simulink model "Symulacja_URA_na_podstawie_aktualnego_TP"  (R2022b)
settings: Solver=VariableStepAuto  StartTime=0.0  StopTime=100  RelTol=1e-3
values from neighbouring files (symbols this model uses):
  TPP = 0.5    [TPP_change.m]
  Ts = TS    [PID_init.m]    (also in Plik_inicjalizujacy_symulacje_predyktora_Smitha.m = 0.01)
undefined symbols (not defined in the file or in its folder): DiscIntNeverNeededParam
settings Model: Creator=hpiet  LastModifiedBy=hpiet
settings DebuggingCC: UnderSpecifiedDimensionMsg=warning

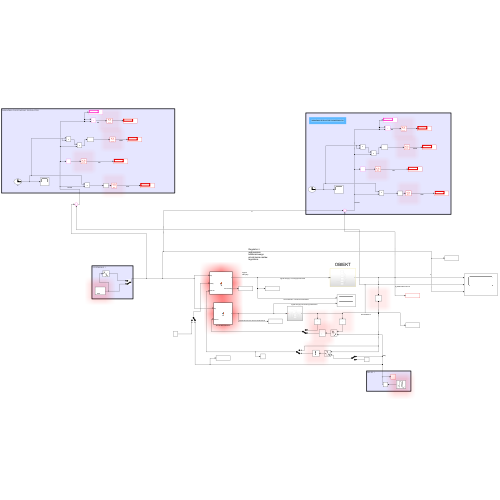
[thumbnail: Simulink's stored preview of the top-level diagram]
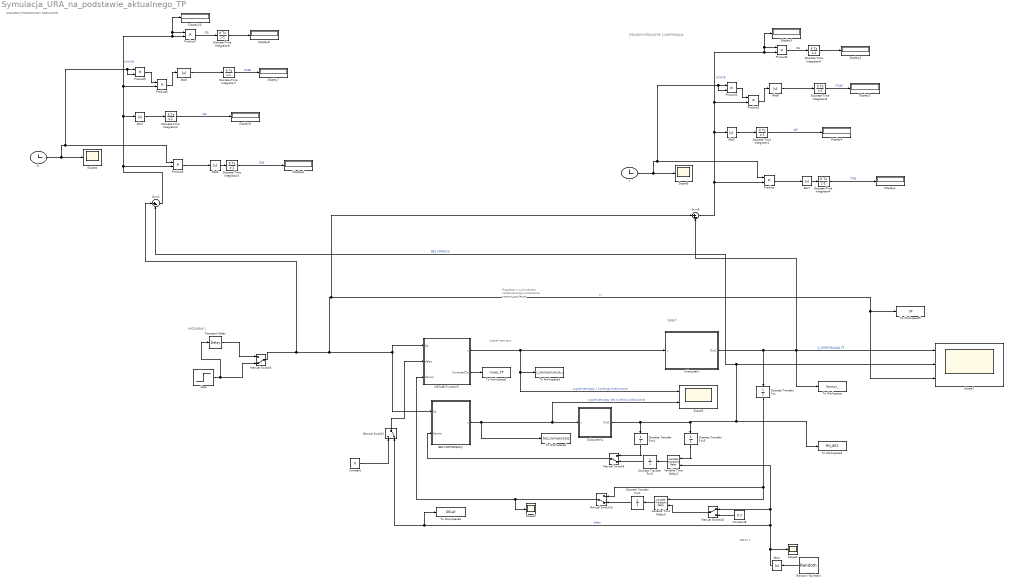
== system Symulacja_URA_na_podstawie_aktualnego_TP ==
  note: WSKAZNIKI REGULATOR Z KOMPENSACJA
  note: WSKAŹNIKI PODSTAWOWY REGULATOR
  note: OBIEKT
  note: DELAY 1
  note: sygnał sterujacy
  note: Regulator z wykonaniem każdorazowego przeliczenia nastaw regulatora
  note: OPÓŹNIENIE 1
  Abs{1..5,7..8} (7 alike) : Abs  SaturateOnIntegerOverflow=off
  BEZ KOMPENSACJI : MATLAB Function  TreatAsAtomicUnit=on  SystemSampleTime=TPP
  Constant : Constant  Value=0
  Constant8 : Constant  Value=0.3
  Discrete Transfer Fcn{,1..4} (5 alike) : DiscreteTransferFcn  Denominator=[1]  SampleTime=TPP
  Discrete-Time Integrator{1..8} (8 alike) : DiscreteIntegrator  SampleTime=Ts  ICPrevOutput=DiscIntNeverNeededParam  ICPrevScaledInput=DiscIntNeverNeededParam
  Display{1..10} (10 alike) : Display
  MATLAB Function3 : MATLAB Function  TreatAsAtomicUnit=on  SystemSampleTime=TPP
  Manual Switch{1,5..6,13} (4 alike) : ManualSwitch  CurrentSetting=0
  Manual Switch16 : ManualSwitch
  Product{,1..7} (8 alike) : Product
  Random Number1 : RandomNumber  Mean=1  Variance=0.0001  SampleTime=TPP
  Scope{1..2,4..5} (4 alike) : Scope
  Scope3 : Scope  NumInputPorts=2
  Scope7 : Scope  NumInputPorts=3
  Step : Step  Time=0  After=25  SampleTime=TPP
  Subsystem : Subsystem
  Subsystem1 : Subsystem
  Sum1 : Sum  Inputs=|+-
  Sum9 : Sum  Inputs=|+-
  To Workspace : ToWorkspace  VariableName=Sensor_  SaveFormat=Timeseries  SampleTime=-1
  To Workspace1 : ToWorkspace  VariableName=nowe_TP  SaveFormat=Timeseries  SampleTime=-1
  To Workspace2 : ToWorkspace  VariableName=PID_BEZ  SaveFormat=Timeseries  SampleTime=-1
  To Workspace3 : ToWorkspace  VariableName=z_kompensacja_u  SaveFormat=Timeseries  SampleTime=-1
  To Workspace4 : ToWorkspace  VariableName=bez_kompensacji  SaveFormat=Timeseries  SampleTime=-1
  To Workspace5 : ToWorkspace  VariableName=SP  SaveFormat=Timeseries  SampleTime=-1
  To Workspace6 : ToWorkspace  VariableName=DELAY  SaveFormat=Timeseries  SampleTime=-1
  Transport Delay : TransportDelay  DelayTime=0
  Variable Time Delay2 : VariableTransportDelay  MaximumDelay=10
  Variable Time Delay5 : VariableTransportDelay  MaximumDelay=10
  t : Clock
  t1 : Clock
  wires:
  Constant8/1 -> Manual Switch16/2
  Random Number1/1 -> Abs1/1
  Manual Switch16/1 -> Variable Time Delay5/2
  Manual Switch13/1 -> MATLAB Function3/3(Sensor), Scope2/1
  MATLAB Function3/1(u) -> Scope3/1, To Workspace3/1, Subsystem/1(u)  "sygnał sterujący z korekcją próbkowania"
  Subsystem/1(Out1) -> Discrete Transfer Fcn/1, Sum9/2, To Workspace/1, Scope7/1  "Z_MODYFIKACJAA TP"
  Variable Time Delay5/1 -> Discrete Transfer Fcn1/1
  Abs1/1 -> Scope1/1, To Workspace6/1, Manual Switch1/2, Manual Switch16/1, Variable Time Delay2/2  "delay"
  Transport Delay/1 -> Manual Switch5/1
  Discrete Transfer Fcn/1 -> Variable Time Delay5/1, Manual Switch13/1
  BEZ KOMPENSACJI/1(u) -> Scope3/2, Subsystem1/1(u), To Workspace4/1  "sygnał sterujący bez korekcji próbkowania"
  Subsystem1/1(Out1) -> To Workspace2/1, Sum1/2, Scope7/2, Discrete Transfer Fcn3/1, Discrete Transfer Fcn4/1  "BEZ KOREKCJI"
  Variable Time Delay2/1 -> Discrete Transfer Fcn2/1
  Discrete Transfer Fcn2/1 -> Manual Switch6/2
  Manual Switch6/1 -> BEZ KOMPENSACJI/2(Sensor)
  Discrete Transfer Fcn3/1 -> Variable Time Delay2/1
  Discrete Transfer Fcn4/1 -> Manual Switch6/1
  Manual Switch1/1 -> MATLAB Function3/2(delay)
  Discrete Transfer Fcn1/1 -> Manual Switch13/2
  Constant/1 -> Manual Switch1/1
  Step/1 -> Transport Delay/1, Manual Switch5/2
  MATLAB Function3/2(CorrectedTp) -> To Workspace1/1
  Product2/1 -> Abs8/1
  Discrete-Time Integrator4/1 -> Display1/1  "ITAE"
  Discrete-Time Integrator5/1 -> Display2/1  "IT2AE"
  Product3/1 -> Discrete-Time Integrator6/1  "ISE"
  Discrete-Time Integrator6/1 -> Display3/1
  Abs7/1 -> Discrete-Time Integrator4/1
  Sum9/1 -> Product/2, Product2/2, Display5/1, Product3/1, Product3/2, Abs5/1  "UCHYB"
  Product1/1 -> Product2/1
  Abs8/1 -> Discrete-Time Integrator5/1
  Abs5/1 -> Discrete-Time Integrator1/1
  Manual Switch5/1 -> Sum1/1, Sum9/1, To Workspace5/1, Scope7/3, MATLAB Function3/1(Sp), BEZ KOMPENSACJI/1(Sp)  "Yr"
  Discrete-Time Integrator1/1 -> Display4/1  "IAE"
  Product/1 -> Abs7/1
  t/1 -> Product1/2, Product1/1, Product/1, Scope5/1
  t1/1 -> Product5/2, Product5/1, Product4/1, Scope4/1
  Product5/1 -> Product6/1
  Abs4/1 -> Discrete-Time Integrator7/1
  Product4/1 -> Abs3/1
  Discrete-Time Integrator8/1 -> Display8/1
  Sum1/1 -> Product4/2, Product6/2, Display10/1, Product7/1, Product7/2, Abs2/1  "UCHYB"
  Product7/1 -> Discrete-Time Integrator8/1  "ISE"
  Discrete-Time Integrator3/1 -> Display6/1  "ITAE"
  Discrete-Time Integrator7/1 -> Display7/1  "IT2AE"
  Abs2/1 -> Discrete-Time Integrator2/1
  Abs3/1 -> Discrete-Time Integrator3/1
  Product6/1 -> Abs4/1
  Discrete-Time Integrator2/1 -> Display9/1  "IAE"

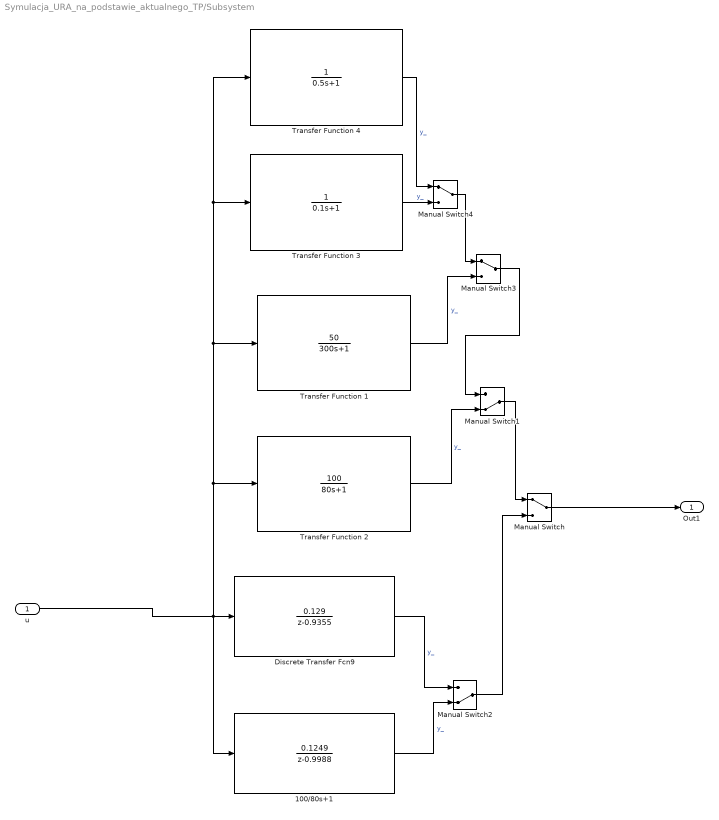
== system Symulacja_URA_na_podstawie_aktualnego_TP/Subsystem ==
  u : Inport
  100/80s+1 : DiscreteTransferFcn  Numerator=[0.1249]  Denominator=[1 -0.9988]  SampleTime=TPP
  Discrete Transfer Fcn9 : DiscreteTransferFcn  Numerator=[0.129]  Denominator=[1 -0.9355]  SampleTime=TPP
  Manual Switch : ManualSwitch
  Manual Switch1 : ManualSwitch  CurrentSetting=0
  Manual Switch2 : ManualSwitch  CurrentSetting=0
  Manual Switch3 : ManualSwitch
  Manual Switch4 : ManualSwitch
  Transfer Function 1 : TransferFcn  Numerator=[50]  Denominator=[300 1]
  Transfer Function 2 : TransferFcn  Numerator=[100]  Denominator=[80 1]
  Transfer Function 3 : TransferFcn  Denominator=[0.1 1]
  Transfer Function 4 : TransferFcn  Denominator=[0.5 1]
  Out1 : Outport
  wires:
  u/1 -> 100/80s+1/1, Discrete Transfer Fcn9/1, Transfer Function 4/1, Transfer Function 3/1, Transfer Function 1/1, Transfer Function 2/1
  Transfer Function 2/1 -> Manual Switch1/2  "y_"
  Manual Switch/1 -> Out1/1
  Transfer Function 1/1 -> Manual Switch3/2  "y_"
  Manual Switch1/1 -> Manual Switch/1
  Manual Switch2/1 -> Manual Switch/2
  Discrete Transfer Fcn9/1 -> Manual Switch2/1  "y_"
  100/80s+1/1 -> Manual Switch2/2  "y_"
  Transfer Function 3/1 -> Manual Switch4/2  "y_"
  Manual Switch3/1 -> Manual Switch1/1
  Transfer Function 4/1 -> Manual Switch4/1  "y_"
  Manual Switch4/1 -> Manual Switch3/1

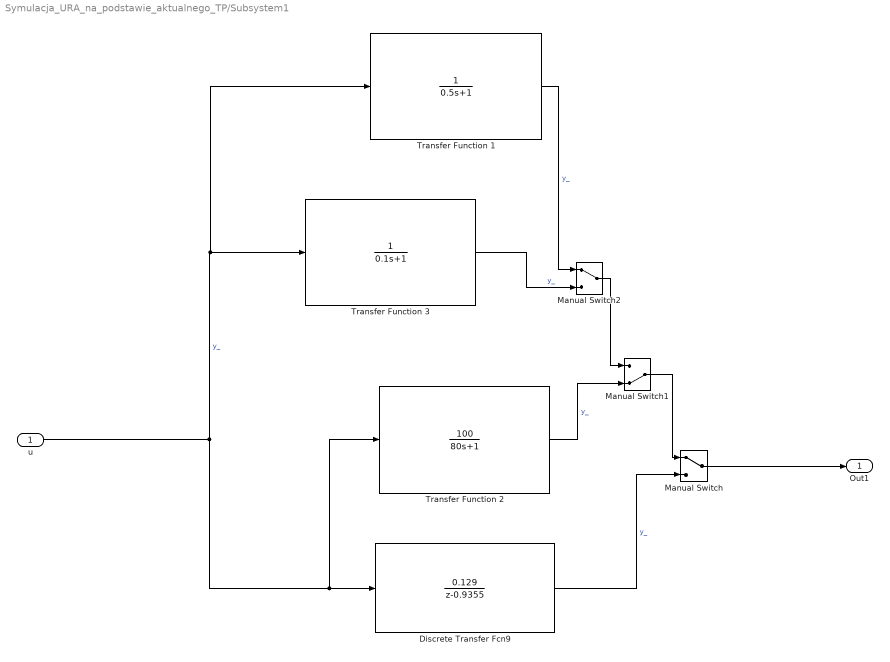
== system Symulacja_URA_na_podstawie_aktualnego_TP/Subsystem1 ==
  u : Inport
  Discrete Transfer Fcn9 : DiscreteTransferFcn  Numerator=[0.129]  Denominator=[1 -0.9355]  SampleTime=TPP
  Manual Switch : ManualSwitch
  Manual Switch1 : ManualSwitch  CurrentSetting=0
  Manual Switch2 : ManualSwitch
  Transfer Function 1 : TransferFcn  Denominator=[0.5 1]
  Transfer Function 2 : TransferFcn  Numerator=[100]  Denominator=[80 1]
  Transfer Function 3 : TransferFcn  Denominator=[0.1 1]
  Out1 : Outport
  wires:
  Discrete Transfer Fcn9/1 -> Manual Switch/2  "y_"
  Transfer Function 2/1 -> Manual Switch1/2  "y_"
  Manual Switch/1 -> Out1/1
  Manual Switch1/1 -> Manual Switch/1
  u/1 -> Transfer Function 1/1, Transfer Function 3/1, Discrete Transfer Fcn9/1, Transfer Function 2/1  "y_"
  Manual Switch2/1 -> Manual Switch1/1
  Transfer Function 3/1 -> Manual Switch2/2  "y_"
  Transfer Function 1/1 -> Manual Switch2/1  "y_"

== matlab function Symulacja_URA_na_podstawie_aktualnego_TP/BEZ KOMPENSACJI ==
  settings: updateMethod=DISCRETE
  data: Sp input; u output; Sensor input
function u= fcn(Sp,Sensor) %wyjscie = funkcja(wejscia)
persistent init e2 e1 u2 u1 ku1 ku2 ke0 ke1 ke2 ;

if isempty(init) %wykonuje się tylko raz
    %NASTAWY WOLNO ZMIENNY
Kp = 0.0975043176181261;
Ki =0.00404938736460088;
Kd = 0.148625801524361;
FCoef = 0.191342781331139;


%NASTAWY SZYBKI
% Kp=0.551095850914855
% Ki=1.79030794942895;
% Kd=0
% FCoef=2.74256026182305

%NASTAWY 0.5s
% Kp=0.352652053728451;
% Ki=0.477399324378819;
% Kd=0;
% FCoef=0.588685123145228;


Ts=0.5; %czas próbki
%TsReal=Ts+delay;


e2=0;
e1=0;
u2=0;
u1=0;

a0 = (1 + FCoef * Ts);
a1 = -(2 + FCoef * Ts);
a2 = 1;

b0=Kp*(1+FCoef * Ts) + Ki*Ts*(1+ FCoef*Ts) + Kd*FCoef;
b1= -(Kp*(2+FCoef*Ts) + Ki*Ts + 2*Kd*FCoef);
b2=Kp + Kd * FCoef;


%TEST
% a0 = (1 + FCoef * TsReal);
% a1 = -(2 + FCoef * TsReal);
% a2 = 1;
% 
% b0=Kp*(1+FCoef * TsReal) + Ki*TsReal*(1+ FCoef*TsReal) + Kd*FCoef;
% b1= -(Kp*(2+FCoef*TsReal) + Ki*TsReal + 2*Kd*FCoef);
% b2=Kp + Kd * FCoef;


%uproszczenie równania
ku1=a1/a0;
ku2=a2/a0;
ke0=b0/a0;
ke1=b1/a0;
ke2=b2/a0;

init=1;
end

e0 = Sp-Sensor;
u0 = -(ku1*u1) - (ku2 * u2) + (ke0*e0) + (ke1*e1) + (ke2*e2);

e2=e1;
e1=e0;
u2=u1;
u1=u0;

u=u0;



end

== matlab function Symulacja_URA_na_podstawie_aktualnego_TP/MATLAB Function3 ==
  settings: updateMethod=DISCRETE
  data: Sp input; u output; delay input; Sensor input; CorrectedTp output
 function [u,CorrectedTp] = PID(Sp,delay,Sensor) %wyjscie = funkcja(wejscia)
persistent init e2 e1 u2 u1 ku1 ku2 ke0 ke1 ke2 actualTp i time_vec previousTp Kp Ki Kd FCoef first_iteration;

if isempty(init) %wykonuje się tylko raz
% Kp =0.00279989495191504;
% Ki =0.0559978990383007;
% Kd = 0;
% FCoef = 100;

%NASTAWY AUTO TUNE SZYBKI 1/0.1s+1!!!
% 
% Kp=0.551095850914855;
% Ki=1.79030794942895;
% Kd=0;
% FCoef=2.74256026182305


%NASTAWY OBIEKT 1/0.5s+1
% 
% Kp=0.352652053728451;
% Ki=0.477399324378819;
% Kd=0;
% FCoef=0.588685123145228;

% Kp=27.6987325006552;
% Ki=0.497836071607621;
% Kd=0;
% FCoef=0.459383555636041;

% 
Kp = 0.0975043176181261;
Ki =0.00404938736460088;
Kd = 0.148625801524361;
FCoef = 0.191342781331139;


%DO SPRAWDZANIA
actualTp=0;
i=0;
time_vec=0;
first_iteration=0;

e2=0;
e1=0;
u2=0;
u1=0;

init=1;
end

%MODYFIKACJA TP
actualTp=i+delay;
time_vec = [time_vec,actualTp];
previousTp=time_vec(end-1);

if(first_iteration==0)
CorrectedTp = actualTp-0.5;
else
    CorrectedTp=actualTp-previousTp
end

 disp('aktualna chwila czasowa')
 disp(actualTp)
% disp('Ostatnia chwila czasowa:')
% disp(previousTp)
disp('TIMESTAMP diff')
disp(CorrectedTp)


if(first_iteration==0)
 a0 = (1 + FCoef * i);
a1 = -(2 + FCoef * i);
a2 = 1;

b0=Kp*(1+FCoef * i) + Ki*i*(1+ FCoef*i) + Kd*FCoef;
b1= -(Kp*(2+FCoef*i) + Ki*i + 2*Kd*FCoef);
b2=Kp + Kd * FCoef;


%uproszczenie równania
ku1=a1/a0;
ku2=a2/a0;
ke0=b0/a0;
ke1=b1/a0;
ke2=b2/a0;

e0 = Sp-Sensor;
%disp(Sensor)
u0 = -(ku1*u1) - (ku2 * u2) + (ke0*e0) + (ke1*e1) + (ke2*e2);

first_iteration=1;
else

a0 = (1 + FCoef * CorrectedTp);
a1 = -(2 + FCoef * CorrectedTp);
a2 = 1;

b0=Kp*(1+FCoef * CorrectedTp) + Ki*CorrectedTp*(1+ FCoef*CorrectedTp) + Kd*FCoef;
b1= -(Kp*(2+FCoef*CorrectedTp) + Ki*CorrectedTp + 2*Kd*FCoef);
b2=Kp + Kd * FCoef;


%uproszczenie równania
ku1=a1/a0;
ku2=a2/a0;
ke0=b0/a0;
ke1=b1/a0;
ke2=b2/a0;

e0 = Sp-Sensor;
%disp(Sensor)
u0 = -(ku1*u1) - (ku2 * u2) + (ke0*e0) + (ke1*e1) + (ke2*e2);
end

%TEST
a0 = (1 + FCoef * CorrectedTp);
a1 = -(2 + FCoef * CorrectedTp);
a2 = 1;

b0=Kp*(1+FCoef * CorrectedTp) + Ki*CorrectedTp*(1+ FCoef*CorrectedTp) + Kd*FCoef;
b1= -(Kp*(2+FCoef*CorrectedTp) + Ki*CorrectedTp + 2*Kd*FCoef);
b2=Kp + Kd * FCoef;


%uproszczenie równania
ku1=a1/a0;
ku2=a2/a0;
ke0=b0/a0;
ke1=b1/a0;
ke2=b2/a0;

e0 = Sp-Sensor;
%disp(Sensor)
u0 = -(ku1*u1) - (ku2 * u2) + (ke0*e0) + (ke1*e1) + (ke2*e2);

e2=e1;
e1=e0;
u2=u1;
u1=u0;

u=u0;
i=i+0.5;

end
